simulink model "Fig143"  (R2014a)
settings: Solver=ode3  StartTime=0  StopTime=1.0  FixedStep=1.25e-6  RelTol=1e-3
undefined symbols (not defined in the file): fdesignblkfcn, gcbh
libraries: commchan3 x1, dspvision x1
(part 1 of 2)
settings Model: Creator=Silage  LastModifiedBy=Silage
settings DebuggingCC: SolverPrmCheckMsg=none  IntegerOverflowMsg=none  ParameterOverflowMsg=none  ParameterPrecisionLossMsg=none

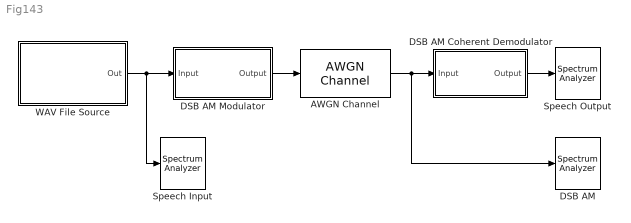
== system Fig143 ==
  AWGN Channel : commchan3/AWGN Channel  InputProcessing=Inherited (this choice will be removed - see release notes)  seed=randseed  noiseMode=Variance from mask  EbNodB=10  EsNodB=10  SNRdB=10  bitsPerSym=1  Ps=1  Tsym=1  variance=0
  "DSB AM " : SpectrumAnalyzer
  DSB AM Coherent Demodulator : Subsystem
  DSB AM Modulator : Subsystem
  Speech Input : SpectrumAnalyzer
  Speech Output : SpectrumAnalyzer
  WAV File Source : Subsystem
  wires:
  AWGN Channel/1 -> "DSB AM "/1, DSB AM Coherent Demodulator/1(Input)
  DSB AM Modulator/1(Output) -> AWGN Channel/1
  WAV File Source/1(Out) -> Speech Input/1, DSB AM Modulator/1(Input)
  DSB AM Coherent Demodulator/1(Output) -> Speech Output/1

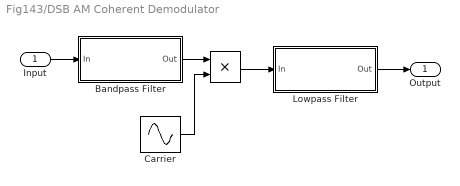
== system Fig143/DSB AM Coherent Demodulator ==
  Input : Inport
  " " : Product  RndMeth=Zero
  Bandpass Filter : Subsystem  DialogController=fdesignblkfcn  InitFcn=fdesignblkfcn(gcbh, {'InitFcn'});  mask(Bandpass Filter){}
      mask help: Design a bandpass filter
      settings: CopyFcn=fdesignblkfcn(gcbh, {'CopyFcn'});
      mask Help: helpview(mapfilelocation('dsp'), 'dspbandpassfilter');
      mask Display: disp('Bandpass');
  Carrier : Sin  Frequency=40000*pi  SampleTime=1.25e-6
  Lowpass Filter : Subsystem  DialogController=fdesignblkfcn  InitFcn=fdesignblkfcn(gcbh, {'InitFcn'});  mask(Lowpass Filter){}
      mask help: Design a lowpass filter
      settings: CopyFcn=fdesignblkfcn(gcbh, {'CopyFcn'});
      mask Help: helpview(mapfilelocation('dsp'), 'dsplowpassfilter');
      mask Display: disp('Lowpass')
  Output : Outport
  wires:
  Carrier/1 -> " "/2
  Input/1 -> Bandpass Filter/1(In)
  Bandpass Filter/1(Out) -> " "/1
  " "/1 -> Lowpass Filter/1(In)
  Lowpass Filter/1(Out) -> Output/1

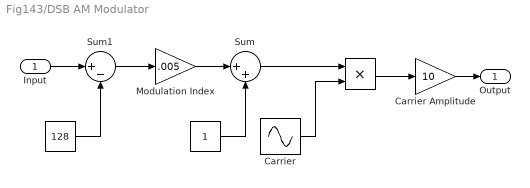
== system Fig143/DSB AM Modulator ==
  Input : Inport
  " " : Product  RndMeth=Zero
  "  " : Constant
  " " : Constant  Value=128
  Carrier : Sin  Frequency=40000*pi  SampleTime=1.25e-6
  Carrier Amplitude : Gain  Gain=10
  Modulation Index : Gain  Gain=.005
  Sum : Sum  Inputs=|++
  Sum1 : Sum  Inputs=|+-
  Output : Outport
  wires:
  Modulation Index/1 -> Sum/1
  "  "/1 -> Sum/2
  Sum/1 -> " "/1
  Carrier/1 -> " "/2
  " "/1 -> Carrier Amplitude/1
  Carrier Amplitude/1 -> Output/1
  " "/1 -> Sum1/2
  Input/1 -> Sum1/1
  Sum1/1 -> Modulation Index/1

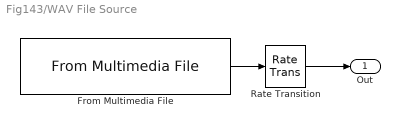
== system Fig143/WAV File Source ==
  From Multimedia File : dspvision/From Multimedia File  inputFilename=C:\Users\Silage\Documents\Digital Communication Simulation using MATLAB and Simulink\Wav Files\Robbie8000.wav  loop=on  numPlays=inf  outputStreams=Audio only  videoDataType=single  audioDataType=uint8  inheritSampleTime=on  userDefinedSampleTime=1/30  noAudioOutput=off  isIntensityVideo=off  fourcc=RGB  colorVideoFormat=Separate color signals  outputEOF=off  dataOrg=Column-major  audioFrameSize=1  computeAudioFrameSize=off  outSamplingMode=Sample based
  Rate Transition : RateTransition  OutPortSampleTime=1.25e-6
  Out : Outport
  wires:
  Rate Transition/1 -> Out/1
  From Multimedia File/1 -> Rate Transition/1

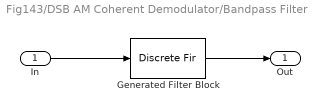
== system Fig143/DSB AM Coherent Demodulator/Bandpass Filter ==
  In : Inport
  Generated Filter Block : DiscreteFir  Tag=BlockMethodSubSystem  Coefficients=[0.00058428545147761271 -0.00013603972061439462 -0.00011636896282705347 -9.6020462205143224e-05 -7.5366977499816384e-05 -5.4398616821042136e-05 -3.3359928242880811e-05 -1.21825025399601e-05 8.8798324694283751e-06 2.983282492642632e-05 5.0302230881884107e-05 7.0141925978349897e-05 8.8804947750613516e-05 0.00010597351091579465 0.00012092505429966959 0.0001332143962958192 0.0001420072975034165 0.00014681783412296651 0.00014681012461509698 0.00014159910371485047 0.00013048344103254325 0.00011332394771424123 8.9695538624002497e-05 5.9848647862890424e-05 2.373914467406133e-05 -1.7883563842208981e-05 -6.4618170917261528e-05 -0.00011516208925794226 -0.00016870118464214958 -0.00022336998971907466 -0.00027808715432663111 -0.00033043556410660091 -0.00037945949040521108 -0.00042175826135881019 -0.00045790841200039412 -0.00048311723324798666 -0.00049724328937429565 -0.0005001227034964116 -0.00048838613191460071 -0.00046201746723236261 -0.00042043008883520846 -0.00036436927040983571 -0.00029387229836124362 -0.00021010575511885154 -0.000114106384858329 -8.0770868382236057e-06 0.00010578170405355445 0.00022437366563305954 0.00034475413897317136 0.0004633549622463255 0.00057688324288477592 0.00068163097895438936 0.00077428997168612333 0.00085134767114980643 0.00090988008556583237 0.00094701412376181106 0.00096067552281337801 0.00094906620868760738 0.00091137089923609823 0.0008471979829586838 0.000757236589068779 0.00064264104749533601 0.00050567666900899321 0.00034897875443561018 0.00017626834690730929 -8.5960380540764089e-06 -0.00020068657002110133 -0.00039538741701700901 -0.00058707641541932553 -0.0007704683161667801 -0.0009407268686043046 -0.0010918672810365641 -0.0012198120995344831 -0.0013202740488554448 -0.0013896267930655194 -0.0014249465839786101 -0.0014245547903956892 -0.0013876027190149634 -0.0013142697579839803 -0.0012056337501668191 -0.0010639166872684575 -0.00089230946188528911 -0.00069500797833708743 -0.00047692829166507479 -0.00024367406532887367 -1.2950626110110863e-06 0.00024376530329731308 0.00048493194542544238 0.00071561448036929116 0.00092948625455645836 0.0011206299785262099 0.0012837843345880524 0.0014144417366224267 0.0015090327570620409 0.0015649851697277896 0.0015808545078739194 0.0015563138874051792 0.001492244624186073 0.0013906404876259659 0.0012546215938304343 0.0010882747797424041 0.00089652467282575073 0.00068516692268667486 0.00046007956508996387 0.00022818356719083268 -4.2492952364307215e-06 -0.00023061246934205732 -0.00044453053937162392 -0.00064035200941146126 -0.00081306164535611372 -0.00095834921866422697 -0.0010728524078561425 -0.0011543508849947823 -0.0012017434951817514 -0.001215012918709586 -0.00119521273288263 -0.0011444629604085703 -0.0010658631577778936 -0.00096336552028121881 -0.0008415636771849684 -0.00070553745644332368 -0.0005606473353832335 -0.00041239067517792946 -0.0002661532716696966 -0.00012704895341909684 3.2577726410366166e-07 0.00011201180935695844 0.00020488297976806205 0.00027667842718456239 0.00032613502871357977 0.00035296060887263496 0.00035791458792444744 0.00034266371035022764 0.00030984334818457082 0.00026273782334080729 0.00020541807613983157 0.00014212623570067457 7.7681414079861698e-05 1.6640499583615531e-05 -3.6483137544916472e-05 -7.7382620348411189e-05 -0.00010260523081910696 -0.00010920876853691594 -9.5134672952163477e-05 -5.9330270866895167e-05 -1.861519559550232e-06 7.6227248936046514e-05 0.00017281382158210539 0.00028475883492743922 0.00040796826935197121 0.00053763117277065239 0.00066833051704171713 0.00079428096759956532 0.00090946886686720505 0.0010079604646059271 0.0010841027287314751 0.0011328307707858417 0.0011498128247163207 0.0011316963836007674 0.0010762238019239923 0.00098243238612231152 0.0008506851299715008 0.00068277272405674154 0.00048183741942089031 0.00025236961085520882 1.1883476117306212e-08 -0.00026848290634638061 -0.00054557838466350061 -0.0008230331680696162 -0.0010923600070892072 -0.0013449075139909149 -0.0015723231983818644 -0.001766835874722225 ...(+14039 chars)]  InputProcessing=Columns as channels (frame based)
  Out : Outport
  wires:
  In/1 -> Generated Filter Block/1
  Generated Filter Block/1 -> Out/1
